simulink model "UpDownDemo1"  (Simulink 5.0)
settings: Solver=ode1  SolverMode=SingleTasking  StartTime=0.0  StopTime=100.0  FixedStep=0.001  RelTol=1e-3
libraries: pci1711 x3
settings Model: LastModifiedBy=cedrics  ExtModeMexFile=rtwinext  ExtModeTrigMode=oneshot  ExtModeTrigDuration=100000  SimulationMode=external  LimitDataPoints=off  BlockReductionOpt=off  BooleanDataType=off  RTWSystemTargetFile=rtwinfbk.tlc  RTWTemplateMakefile=winfbktmf  RTWOptions="-aCCOptimize=1 -aEnforceIntegerDowncast=1 -aExtMode=1 -aFoldNonRolledExpr=1 -aForceParamTrailComments=0 -aGenerateComments=1 -aGenerateReport=0 -aIncDataTypeInIds=0 -aIncHierarchyInIds=0 -aInlineInvariantSignals=0 -aInlineParameters=0 -aInlinedPrmAccess=\"Literals\" -aLocalBlockOutputs=1 -aMaxRTWIdLen=31 -aPrefixModelToSubsysFcnNames=1 -aRTWVerbose=1 -aRebuildAll=0 -aRollThreshold=5 -aShowEliminatedStatements=1"

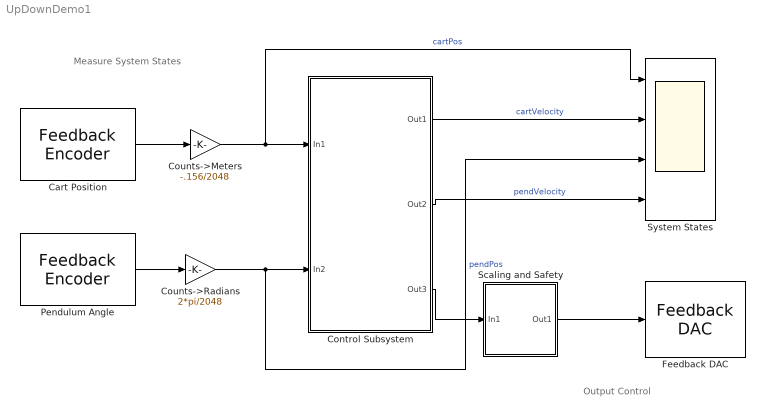
== system UpDownDemo1 ==
  note: Measure System States
  note: Output Control
  "Cart Position " : pci1711/Advantech  PCI1711 I//O Board Lib/Feedback Encoder   channel=0  offset=0  tsamp=0.001  hwAccess=on
  Control Subsystem : Subsystem
  Counts->Meters : Gain  Gain=-.156/2048  SaturateOnIntegerOverflow=on
  Counts->Radians : Gain  Gain=2*pi/2048  SaturateOnIntegerOverflow=on
  Feedback DAC : pci1711/Advantech  PCI1711 I//O Board Lib/Feedback DAC  channel=0  range=0  tsamp=0.001  hwAccess=on
  "Pendulum Angle " : pci1711/Advantech  PCI1711 I//O Board Lib/Feedback Encoder   channel=1  offset=-1024  tsamp=0.001  hwAccess=on
  Scaling and Safety : Subsystem
  System States : Scope  NumInputPorts=4
      settings: TimeRange=100  YMin=-0.175~-0.9~-0.5~-12.5  YMax=0.175~0.8~6~12.5  SampleInput=on  SampleTime=0.01
  wires:
  Control Subsystem/3(Out3) -> Scaling and Safety/1(In1)
  "Cart Position "/1 -> Counts->Meters/1
  Counts->Meters/1 -> System States/1, Control Subsystem/1(In1)  "cartPos"
  "Pendulum Angle "/1 -> Counts->Radians/1
  Counts->Radians/1 -> System States/3, Control Subsystem/2(In2)  "pendPos"
  Scaling and Safety/1(Out1) -> Feedback DAC/1
  Control Subsystem/1(Out1) -> System States/2  "cartVelocity"
  Control Subsystem/2(Out2) -> System States/4  "pendVelocity"

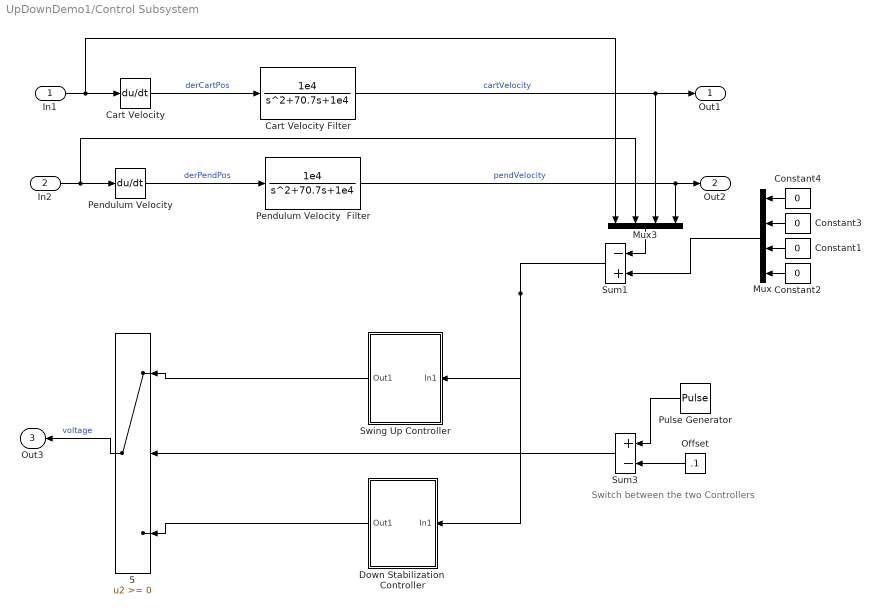
== system UpDownDemo1/Control Subsystem ==
  note: Switch between the
      | two Controllers
  In1 : Inport
  In2 : Inport  Port=2
  5 : Switch  Orientation=left  SaturateOnIntegerOverflow=on  InputSameDT=on
  Cart Velocity : Derivative
  Cart Velocity Filter : TransferFcn  Numerator=[1e4]  Denominator=[1 70.7 1e4]
  Constant{1..4} (4 alike) : Constant  Orientation=left  Value=0
  Down Stabilization  Controller : Subsystem  Orientation=left
  Mux : Mux  Orientation=left
  Mux3 : Mux  Orientation=down
  Offset : Constant  Orientation=left  Value=.1
  Pendulum Velocity : Derivative
  Pendulum Velocity  Filter : TransferFcn  Numerator=[1e4]  Denominator=[1 70.7 1e4]
  Pulse Generator : DiscretePulseGenerator  Orientation=left  PulseType=Time based  Period=30  PulseWidth=70
  Sum1 : Sum  Orientation=left  Inputs=-+  SaturateOnIntegerOverflow=on  InputSameDT=on
  Sum3 : Sum  Orientation=left  Inputs=+-  SaturateOnIntegerOverflow=on  InputSameDT=on
  Swing Up Controller : Subsystem  Orientation=left
  Out1 : Outport
  Out2 : Outport  Port=2
  Out3 : Outport  Orientation=left  Port=3
  wires:
  Swing Up Controller/1(Out1) -> 5/1
  Pulse Generator/1 -> Sum3/1
  Offset/1 -> Sum3/2
  Sum3/1 -> 5/2
  Down Stabilization  Controller/1(Out1) -> 5/3
  Cart Velocity/1 -> Cart Velocity Filter/1  "derCartPos"
  Pendulum Velocity/1 -> Pendulum Velocity  Filter/1  "derPendPos"
  Constant2/1 -> Mux/4
  Constant1/1 -> Mux/3
  Mux/1 -> Sum1/2
  Mux3/1 -> Sum1/1
  Cart Velocity Filter/1 -> Mux3/3, Out1/1  "cartVelocity"
  Pendulum Velocity  Filter/1 -> Mux3/4, Out2/1  "pendVelocity"
  Constant3/1 -> Mux/2
  Constant4/1 -> Mux/1
  Sum1/1 -> Down Stabilization  Controller/1(In1), Swing Up Controller/1(In1)
  In1/1 -> Cart Velocity/1, Mux3/1
  In2/1 -> Pendulum Velocity/1, Mux3/2
  5/1 -> Out3/1  "voltage"

== system UpDownDemo1/Scaling and Safety ==
  In1 : Inport
  -1 : Gain  Gain=-1  SaturateOnIntegerOverflow=on
  Saturation : Saturate  UpperLimit=2.5  LowerLimit=-2.5
  Out1 : Outport
  wires:
  Saturation/1 -> Out1/1
  In1/1 -> -1/1
  -1/1 -> Saturation/1  "actual LoadPosition"

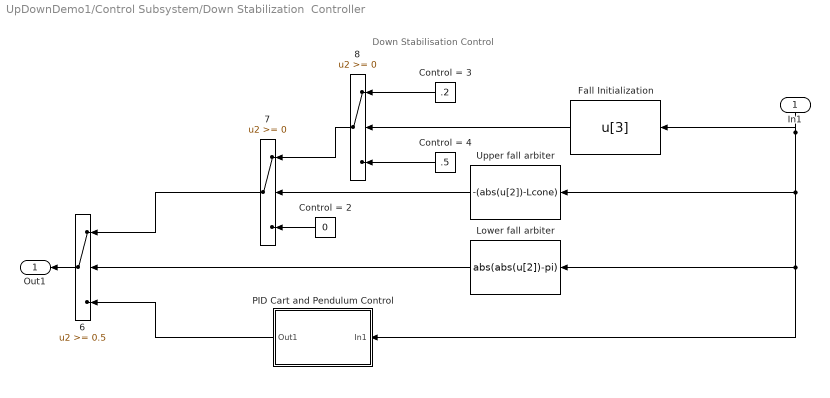
== system UpDownDemo1/Control Subsystem/Down Stabilization  Controller ==
  note: Down Stabilisation Control
  In1 : Inport  Orientation=down
  6 : Switch  Orientation=left  Threshold=0.5  SaturateOnIntegerOverflow=on  InputSameDT=on
  7 : Switch  Orientation=left  SaturateOnIntegerOverflow=on  InputSameDT=on
  8 : Switch  Orientation=left  SaturateOnIntegerOverflow=on  InputSameDT=on
  Control = 2 : Constant  Orientation=left  Value=0
  Control = 3 : Constant  Orientation=left  Value=.2
  Control = 4 : Constant  Orientation=left  Value=.5
  Fall Initialization : Fcn  Orientation=left  Expr=u[3]
      mask Type: ZONE
      mask Description: ZONE
      mask Display: plot(0,0,100,100,[40,60,80,83,80,60,40,20,17,20,40],[89,89,80,70,60,51,51,60,69,80,90],[83,50,17],[70,8,68])
  Lower fall arbiter : Fcn  Orientation=left  Expr=abs(abs(u[2])-pi)
      mask Type: ZONE
      mask Description: ZONE
      mask Display: plot(0,0,100,100,[40,60,80,83,80,60,40,20,17,20,40],[89,89,80,70,60,51,51,60,69,80,90],[83,50,17],[70,8,68])
  PID Cart and Pendulum Control : Subsystem  Orientation=left
      mask Type: linear
      mask Display: plot(0,0,100,100,[40,30,20],[87,85,80],[46,54,54,46,46],[90,90,80,80,90],[46,45,45,46,54,55,55,54,46],[78,80,90,91,91,90,80,78,78],[51,51,49,49],[78,10,10,78],[90,80,70,60],[70,80,85,88],[20,10],[80,70],[20,20,15],[73,80,80],[85,80,80],[80,80,74])
  Upper fall arbiter : Fcn  Orientation=left  Expr=-(abs(u[2])-Lcone)  mask(ZONE){Lcone=0.3}
      mask prompts: Lcone "Cone Width"
      mask help: ZONE
      mask Display: plot(0,0,100,100,[40,60,80,83,80,60,40,20,17,20,40],[89,89,80,70,60,51,51,60,69,80,90],[83,50,17],[70,8,68])
  Out1 : Outport  Orientation=left
  wires:
  Control = 2/1 -> 7/3
  Lower fall arbiter/1 -> 6/2
  PID Cart and Pendulum Control/1(Out1) -> 6/3
  7/1 -> 6/1
  Upper fall arbiter/1 -> 7/2
  8/1 -> 7/1
  Control = 3/1 -> 8/1
  Control = 4/1 -> 8/3
  Fall Initialization/1 -> 8/2
  In1/1 -> Lower fall arbiter/1, PID Cart and Pendulum Control/1(In1), Upper fall arbiter/1, Fall Initialization/1
  6/1 -> Out1/1

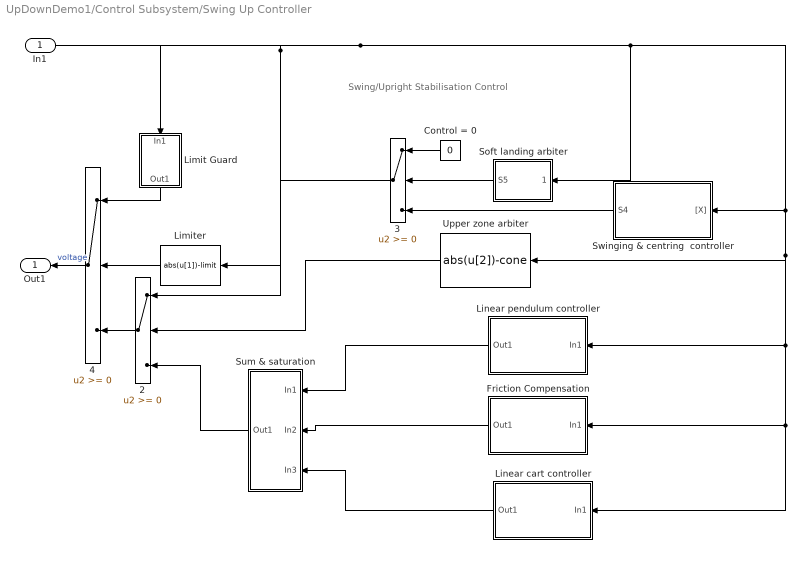
== system UpDownDemo1/Control Subsystem/Swing Up Controller ==
  note: Swing/Upright Stabilisation Control
  In1 : Inport
  2 : Switch  Orientation=left  SaturateOnIntegerOverflow=on  InputSameDT=on
  3 : Switch  Orientation=left  SaturateOnIntegerOverflow=on  InputSameDT=on
  4 : Switch  Orientation=left  SaturateOnIntegerOverflow=on  InputSameDT=on
  Control = 0 : Constant  Orientation=left  Value=0
  Friction Compensation : Subsystem  Orientation=left  mask(linear){frictionCompNeg=.1, frictionCompPos=.1}
      mask prompts: frictionCompNeg "Friction Compensation Magnitude in Negative Direction"; frictionCompPos "Friction Compensation Magnitude in Positive Direction"
      mask Display: plot(0,0,100,100,[40,30,20],[87,85,80],[46,54,54,46,46],[90,90,80,80,90],[46,45,45,46,54,55,55,54,46],[78,80,90,91,91,90,80,78,78],[51,51,49,49],[78,10,10,78],[90,80,70,60],[70,80,85,88],[20,10],[80,70],[20,20,15],[73,80,80],[85,80,80],[80,80,74])
  Limit Guard : Subsystem  Orientation=down  mask{umax2=.5}
      mask prompts: umax2 "maximal force"
      mask Display: plot(0,0,100,100,[20,40,40,20,20],[60,60,49,49,60],[56,59,40],[58,55,55],[56,59],[52,55],[38,13,13],[39,39,46],[46,13],[46,46],[23,23,24,22,24,24,22,23],[47,45,49,48,48,46,47,49],[36,35,34,34,37,34,36,35,36,37,35,34,35],[49,48,46,49,48,47,45,47,48,46,46,47,49],[22,22,24,24],[46,49,48,47])
  Limiter : Fcn  Orientation=left  Expr=abs(u[1])-limit  mask{limit=0.3}
      mask prompts: limit "Rail mg - rail limit"
      mask Display: plot(0,0,100,100,[10,90,90,10],[52,52,50,50],[30,30],[52,60],[70,68,68,70,70],[60,60,52,52,60],[30,32,32,30],[52,52,60,60])
  Linear cart controller : Subsystem  Orientation=left  mask(linear){K1=-7, K3=-4}
      mask prompts: K1 "K1  - position  feedback"; K3 "K3  -  velocity  feedback"
      mask Display: plot(0,0,100,100,[40,30,20],[87,85,80],[46,54,54,46,46],[90,90,80,80,90],[46,45,45,46,54,55,55,54,46],[78,80,90,91,91,90,80,78,78],[51,51,49,49],[78,10,10,78],[90,80,70,60],[70,80,85,88],[20,10],[80,70],[20,20,15],[73,80,80],[85,80,80],[80,80,74])
  Linear pendulum controller : Subsystem  Orientation=left  mask(linear){K2=50, K4=3.5}
      mask prompts: K2 "K2  - angle  feedback"; K4 "K4  - angular velocity  feedback"
      mask Display: plot(0,0,100,100,[40,30,20],[87,85,80],[46,54,54,46,46],[90,90,80,80,90],[46,45,45,46,54,55,55,54,46],[78,80,90,91,91,90,80,78,78],[51,51,49,49],[78,10,10,78],[90,80,70,60],[70,80,85,88],[20,10],[80,70],[20,20,15],[73,80,80],[85,80,80],[80,80,74])
  Soft landing arbiter : Subsystem  Orientation=left  mask(Soft landing){k=8.7, R=0.35}
      mask prompts: k "k coefficient"; R "R value"
      mask help: Soft landing
      mask Display: plot(0,0,100,100,[14,20,20,14,14],[20,20,8,8,20],[40,35,35,40,40],[39,40,51,51,40],[60,55,55,56,60,60],[70,70,60,60,60,71],[74,74,80,80,74],[80,91,91,80,80])
  Sum & saturation : Subsystem  Orientation=left  mask{umax1=2.5}
      mask prompts: umax1 "max control"
  Swinging & centring  controller : Subsystem  Orientation=left  mask(swing){umax=1, alfa=2.2, beta=.4, gamma=0.}
      mask prompts: umax "maximal control umax"; alfa "ALPHA - centering cart factor related to position"; beta "BETA - centering cart factor related to velocity"; gamma "GAMMA - centering cart factor related to + - pi/2 angle"
      mask help: swing
      mask Display: plot(0,0,100,100,[20,20],[12,87],[93,90,90,93,7],[50,46,54,50,50],[20,22,18,20],[87,80,80,88],[80,80,75,75,71,71,65,65,60,60,49,49,40,40,20],[50,40,40,60,60,50,50,80,80,20,21,80,80,21,20])
  Upper zone arbiter : Fcn  Orientation=left  Expr=abs(u[2])-cone  mask(ZONE){cone=.3}
      mask prompts: cone "Stab.zone - width of stabilization zone [rad]"
      mask help: ZONE
      mask Display: plot(0,0,100,100,[40,60,80,83,80,60,40,20,17,20,40],[89,89,80,70,60,51,51,60,69,80,90],[83,50,17],[70,8,68])
  Out1 : Outport  Orientation=left
  wires:
  Limit Guard/1(Out1) -> 4/1
  3/1 -> 2/1
  Swinging & centring  controller/1(S4) -> 3/3
  2/1 -> 4/3
  Soft landing arbiter/1(S5) -> 3/2
  Limiter/1 -> 4/2
  Control = 0/1 -> 3/1
  Linear pendulum controller/1(Out1) -> Sum & saturation/1(In1)
  Upper zone arbiter/1 -> 2/2
  Sum & saturation/1(Out1) -> 2/3
  Friction Compensation/1(Out1) -> Sum & saturation/2(In2)
  Linear cart controller/1(Out1) -> Sum & saturation/3(In3)
  In1/1 -> Soft landing arbiter/1((x1,x2,x3,x4)), Upper zone arbiter/1, Linear pendulum controller/1(In1), Friction Compensation/1(In1), Linear cart controller/1(In1), Swinging & centring  controller/1("[X]"), Limiter/1, Limit Guard/1(In1)
  4/1 -> Out1/1  "voltage"

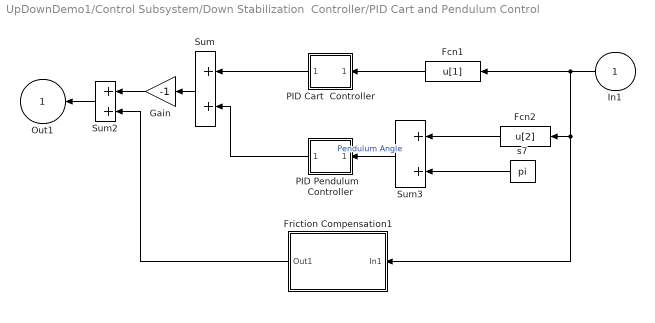
== system UpDownDemo1/Control Subsystem/Down Stabilization  Controller/PID Cart and Pendulum Control ==
  In1 : Inport  Orientation=left
  Fcn1 : Fcn  Orientation=left  Expr=u[1]
  Fcn2 : Fcn  Orientation=left  Expr=u[2]
  Friction Compensation1 : Subsystem  Orientation=left  mask(linear){frictionCompNeg=.1, frictionCompPos=.1}
      mask prompts: frictionCompNeg "Friction Compensation Magnitude in Negative Direction"; frictionCompPos "Friction Compensation Magnitude in Positive Direction"
      mask Display: plot(0,0,100,100,[40,30,20],[87,85,80],[46,54,54,46,46],[90,90,80,80,90],[46,45,45,46,54,55,55,54,46],[78,80,90,91,91,90,80,78,78],[51,51,49,49],[78,10,10,78],[90,80,70,60],[70,80,85,88],[20,10],[80,70],[20,20,15],[73,80,80],[85,80,80],[80,80,74])
  Gain : Gain  Orientation=left  Gain=-1  SaturateOnIntegerOverflow=on
  PID Cart  Controller : Subsystem  Orientation=left  mask(PID Controller){@1=-10, @2=-2, @3=-2}
      mask prompts: @1 "Proportional:"; @2 "Integral"; @3 "Derivative:"
      mask help:
      | Enter expressions for proportional, integral, and derivative terms.
      | P+I/s+Ds
      mask init:
      | P=@1; I=@2; D=@3;
      mask Help: This block implements a PID controller where parameters are entered for the Proportional, Integral and Derivative terms. Unmask this block to see how it works. The derivative term is implemented using a true derivative block.
      mask Display: disp('PID')
  PID Pendulum   Controller : Subsystem  Orientation=left  mask(PID Controller){@1=5, @2=0, @3=0}
      mask prompts: @1 "Proportional:"; @2 "Integral"; @3 "Derivative:"
      mask help:
      | Enter expressions for proportional, integral, and derivative terms.
      | P+I/s+Ds
      mask init:
      | P=@1; I=@2; D=@3;
      mask Help: This block implements a PID controller where parameters are entered for the Proportional, Integral and Derivative terms. Unmask this block to see how it works. The derivative term is implemented using a true derivative block.
      mask Display: disp('PID')
  Sum : Sum  Orientation=left  SaturateOnIntegerOverflow=on  InputSameDT=on
  Sum2 : Sum  Orientation=left  SaturateOnIntegerOverflow=on  InputSameDT=on
  Sum3 : Sum  Orientation=left  SaturateOnIntegerOverflow=on  InputSameDT=on
  s7 : Constant  Orientation=left  Value=pi
  Out1 : Outport  Orientation=left  InitialOutput=0
  wires:
  s7/1 -> Sum3/2
  Fcn1/1 -> PID Cart  Controller/1(In_1)
  Sum3/1 -> PID Pendulum   Controller/1(In_1)  "Pendulum Angle"
  Fcn2/1 -> Sum3/1
  In1/1 -> Fcn1/1, Fcn2/1, Friction Compensation1/1(In1)
  Sum/1 -> Gain/1
  PID Pendulum   Controller/1(Out_1) -> Sum/2
  PID Cart  Controller/1(Out_1) -> Sum/1
  Gain/1 -> Sum2/1
  Sum2/1 -> Out1/1
  Friction Compensation1/1(Out1) -> Sum2/2

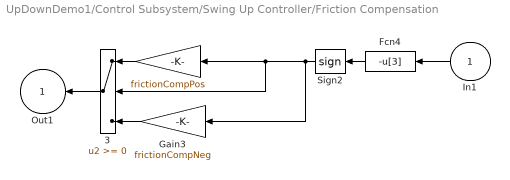
== system UpDownDemo1/Control Subsystem/Swing Up Controller/Friction Compensation ==
  In1 : Inport  Orientation=left
  " " : Gain  Orientation=left  Gain=frictionCompPos  SaturateOnIntegerOverflow=on
  3 : Switch  Orientation=left  SaturateOnIntegerOverflow=on  InputSameDT=on
  Fcn4 : Fcn  Orientation=left  Expr=-u[3]
  Gain3 : Gain  Orientation=left  Gain=frictionCompNeg  SaturateOnIntegerOverflow=on
  Sign2 : Signum  Tag=T  Orientation=left
  Out1 : Outport  Orientation=left  InitialOutput=0
  wires:
  Fcn4/1 -> Sign2/1
  In1/1 -> Fcn4/1
  " "/1 -> 3/1
  Gain3/1 -> 3/3
  Sign2/1 -> Gain3/1, " "/1, 3/2
  3/1 -> Out1/1

== system UpDownDemo1/Control Subsystem/Swing Up Controller/Limit Guard ==
  In1 : Inport
  Fcn : Fcn  Expr=u[1]
  Gain : Gain  Gain=umax2  SaturateOnIntegerOverflow=on
  Sign : Signum
  Out1 : Outport  InitialOutput=0
  wires:
  Sign/1 -> Gain/1
  Gain/1 -> Out1/1
  Fcn/1 -> Sign/1
  In1/1 -> Fcn/1

== system UpDownDemo1/Control Subsystem/Swing Up Controller/Linear cart controller ==
  In1 : Inport  Orientation=left
  Fcn1 : Fcn  Orientation=left  Expr=K1*u[1]
  Fcn2 : Fcn  Orientation=left  Expr=K3*u[3]
  Sum : Sum  Orientation=left  SaturateOnIntegerOverflow=on  InputSameDT=on
  Out1 : Outport  Orientation=left  InitialOutput=0
  wires:
  Fcn1/1 -> Sum/1
  Fcn2/1 -> Sum/2
  Sum/1 -> Out1/1
  In1/1 -> Fcn1/1, Fcn2/1

== system UpDownDemo1/Control Subsystem/Swing Up Controller/Linear pendulum controller ==
  In1 : Inport  Orientation=left
  Fcn2 : Fcn  Orientation=left  Expr=K4*u[4]
  Fcn3 : Fcn  Orientation=left  Expr=K2*atan2(sin(u[2]),cos(u[2]))
  Sum : Sum  Orientation=left  SaturateOnIntegerOverflow=on  InputSameDT=on
  Out1 : Outport  Orientation=left  InitialOutput=0
  wires:
  Sum/1 -> Out1/1
  Fcn2/1 -> Sum/2
  In1/1 -> Fcn2/1, Fcn3/1
  Fcn3/1 -> Sum/1

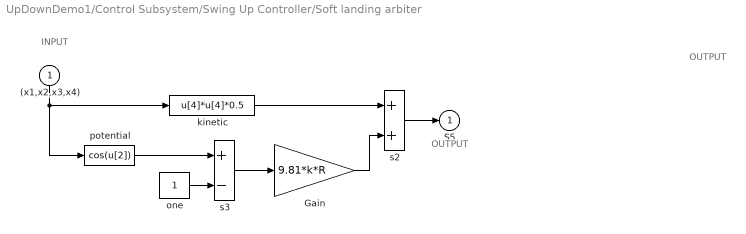
== system UpDownDemo1/Control Subsystem/Swing Up Controller/Soft landing arbiter ==
  note: OUTPUT
  note: OUTPUT
  note: INPUT
  (x1,x2,x3,x4) : Inport  Orientation=down
  Gain : Gain  Gain=9.81*k*R  SaturateOnIntegerOverflow=on
  kinetic : Fcn  Expr=u[4]*u[4]*0.5
  "one " : Constant
  potential : Fcn  Expr=cos(u[2])
  s2 : Sum  SaturateOnIntegerOverflow=on  InputSameDT=on
  s3 : Sum  Inputs=+-  SaturateOnIntegerOverflow=on  InputSameDT=on
  S5 : Outport  InitialOutput=0
  wires:
  potential/1 -> s3/1
  "one "/1 -> s3/2
  kinetic/1 -> s2/1
  s3/1 -> Gain/1
  Gain/1 -> s2/2
  (x1,x2,x3,x4)/1 -> potential/1, kinetic/1
  s2/1 -> S5/1

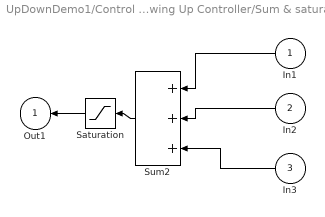
== system UpDownDemo1/Control Subsystem/Swing Up Controller/Sum & saturation ==
  In1 : Inport  Orientation=left
  In2 : Inport  Orientation=left  Port=2
  In3 : Inport  Orientation=left  Port=3
  Saturation : Saturate  Orientation=left  UpperLimit=umax1  LowerLimit=-umax1
  Sum2 : Sum  Orientation=left  Inputs=+++  SaturateOnIntegerOverflow=on  InputSameDT=on
  Out1 : Outport  Orientation=left  InitialOutput=0
  wires:
  In2/1 -> Sum2/2
  Saturation/1 -> Out1/1
  In1/1 -> Sum2/1
  Sum2/1 -> Saturation/1
  In3/1 -> Sum2/3

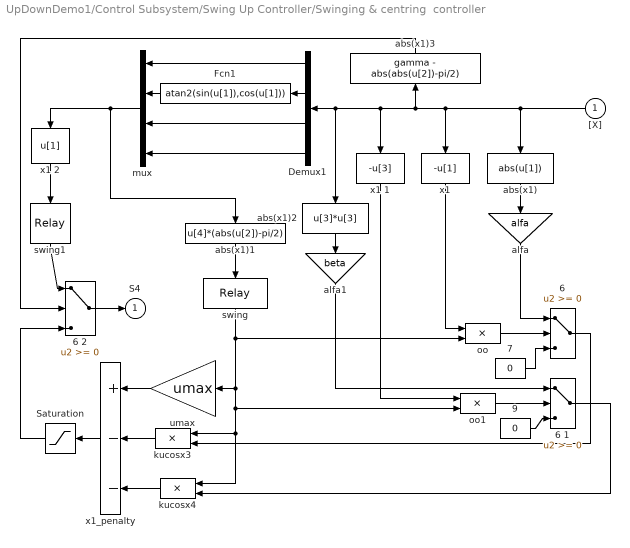
== system UpDownDemo1/Control Subsystem/Swing Up Controller/Swinging & centring  controller ==
  "[X]" : Inport  Orientation=left
  "6 " : Switch  SaturateOnIntegerOverflow=on  InputSameDT=on
  6 1 : Switch  SaturateOnIntegerOverflow=on  InputSameDT=on
  6 2 : Switch  SaturateOnIntegerOverflow=on  InputSameDT=on
  7 : Constant  Value=0
  9 : Constant  Value=0
  Demux1 : Demux  Orientation=left
  Fcn1 : Fcn  Orientation=left  Expr=atan2(sin(u[1]),cos(u[1]))
  Saturation : Saturate  Orientation=left  UpperLimit=umax  LowerLimit=-umax
  abs(x1) : Fcn  Orientation=down  Expr=abs(u[1])
  abs(x1)1 : Fcn  Orientation=down  Expr=u[4]*(abs(u[2])-pi/2)
  abs(x1)2 : Fcn  Orientation=down  Expr=u[3]*u[3]
  abs(x1)3 : Fcn  Orientation=up  Expr=gamma - abs(abs(u[2])-pi/2)
  alfa : Gain  Orientation=down  Gain=alfa  SaturateOnIntegerOverflow=on
  alfa1 : Gain  Orientation=down  Gain=beta  SaturateOnIntegerOverflow=on
  kucosx3 : Product  Orientation=left  SaturateOnIntegerOverflow=on  InputSameDT=on
  kucosx4 : Product  Orientation=left  SaturateOnIntegerOverflow=on  InputSameDT=on
  mux : Mux  Orientation=left
  oo : Product  SaturateOnIntegerOverflow=on  InputSameDT=on
  oo1 : Product  SaturateOnIntegerOverflow=on  InputSameDT=on
  swing : Relay  Orientation=down  OffOutputValue=-1
  swing1 : Relay  Orientation=down  OffOutputValue=-1
  umax : Gain  Orientation=left  Gain=umax  SaturateOnIntegerOverflow=on
  "x1 " : Fcn  Orientation=down  Expr=-u[1]
  x1 1 : Fcn  Orientation=down  Expr=-u[3]
  x1 2 : Fcn  Orientation=down  Expr=u[1]
  x1_penalty : Sum  Orientation=left  Inputs=+--  SaturateOnIntegerOverflow=on  InputSameDT=on
  S4 : Outport  InitialOutput=0
  wires:
  abs(x1)3/1 -> 6 2/2
  Demux1/4 -> mux/4
  Demux1/3 -> mux/3
  Demux1/1 -> mux/1
  Fcn1/1 -> mux/2
  Demux1/2 -> Fcn1/1
  x1_penalty/1 -> Saturation/1
  umax/1 -> x1_penalty/1
  kucosx3/1 -> x1_penalty/2
  oo/1 -> "6 "/2
  "6 "/1 -> kucosx3/2
  abs(x1)/1 -> alfa/1
  abs(x1)1/1 -> swing/1
  "[X]"/1 -> "x1 "/1, x1 1/1, Demux1/1, abs(x1)2/1, abs(x1)3/1, abs(x1)/1
  swing/1 -> umax/1, oo1/2, kucosx3/1, kucosx4/1, oo/2
  alfa/1 -> "6 "/1
  "x1 "/1 -> oo/1
  oo1/1 -> 6 1/2
  alfa1/1 -> 6 1/1
  x1 1/1 -> oo1/1
  abs(x1)2/1 -> alfa1/1
  kucosx4/1 -> x1_penalty/3
  6 1/1 -> kucosx4/2
  7/1 -> "6 "/3
  9/1 -> 6 1/3
  6 2/1 -> S4/1
  Saturation/1 -> 6 2/3
  x1 2/1 -> swing1/1
  mux/1 -> abs(x1)1/1, x1 2/1
  swing1/1 -> 6 2/1

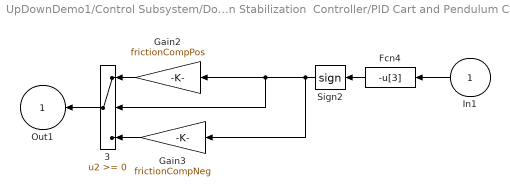
== system UpDownDemo1/Control Subsystem/Down Stabilization  Controller/PID Cart and Pendulum Control/Friction Compensation1 ==
  In1 : Inport  Orientation=left
  3 : Switch  Orientation=left  SaturateOnIntegerOverflow=on  InputSameDT=on
  Fcn4 : Fcn  Orientation=left  Expr=-u[3]
  Gain2 : Gain  Orientation=left  Gain=frictionCompPos  SaturateOnIntegerOverflow=on
  Gain3 : Gain  Orientation=left  Gain=frictionCompNeg  SaturateOnIntegerOverflow=on
  Sign2 : Signum  Tag=T  Orientation=left
  Out1 : Outport  Orientation=left  InitialOutput=0
  wires:
  3/1 -> Out1/1
  Sign2/1 -> 3/2, Gain2/1, Gain3/1
  Gain3/1 -> 3/3
  Gain2/1 -> 3/1
  In1/1 -> Fcn4/1
  Fcn4/1 -> Sign2/1

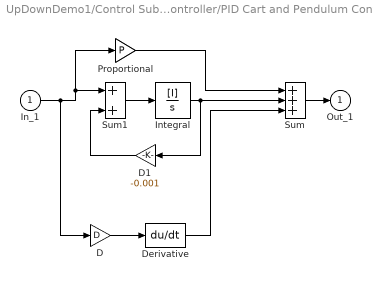
== system UpDownDemo1/Control Subsystem/Down Stabilization  Controller/PID Cart and Pendulum Control/PID Cart  Controller ==
  In_1 : Inport
  D : Gain  Gain=D  SaturateOnIntegerOverflow=on
  D1 : Gain  Orientation=left  Gain=-0.001  SaturateOnIntegerOverflow=on
  Derivative : Derivative
  Integral : TransferFcn  Numerator=[I]  Denominator=[1 0]
  Proportional : Gain  Gain=P  SaturateOnIntegerOverflow=on
  Sum : Sum  Inputs=+++  SaturateOnIntegerOverflow=on  InputSameDT=on
  Sum1 : Sum  SaturateOnIntegerOverflow=on  InputSameDT=on
  Out_1 : Outport  InitialOutput=0
  wires:
  In_1/1 -> D/1, Proportional/1, Sum1/1
  Proportional/1 -> Sum/1
  D/1 -> Derivative/1
  Derivative/1 -> Sum/3
  Sum/1 -> Out_1/1
  Sum1/1 -> Integral/1
  Integral/1 -> Sum/2, D1/1
  D1/1 -> Sum1/2

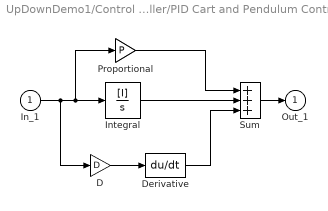
== system UpDownDemo1/Control Subsystem/Down Stabilization  Controller/PID Cart and Pendulum Control/PID Pendulum   Controller ==
  In_1 : Inport
  D : Gain  Gain=D  SaturateOnIntegerOverflow=on
  Derivative : Derivative
  Integral : TransferFcn  Numerator=[I]  Denominator=[1 0]
  Proportional : Gain  Gain=P  SaturateOnIntegerOverflow=on
  Sum : Sum  Inputs=+++  SaturateOnIntegerOverflow=on  InputSameDT=on
  Out_1 : Outport  InitialOutput=0
  wires:
  Proportional/1 -> Sum/1
  Integral/1 -> Sum/2
  Derivative/1 -> Sum/3
  In_1/1 -> Proportional/1, Integral/1, D/1
  Sum/1 -> Out_1/1
  D/1 -> Derivative/1
